simulink model "stoppuhr"  (R2021a)
settings: Solver=ode3  StartTime=0.0  StopTime=10.0  FixedStep=0.01  RelTol=1e-3
settings Model: Creator=Oceaner  LastModifiedBy=Oceaner

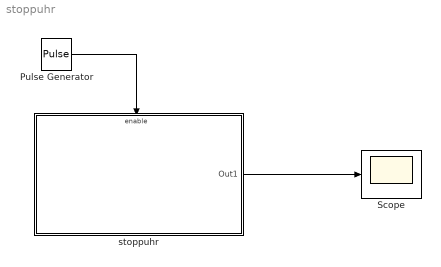
== system stoppuhr ==
  " stoppuhr" : Subsystem  TreatAsAtomicUnit=on
  Pulse Generator : DiscretePulseGenerator  PulseType=Time based  PulseWidth=50
  Scope : Scope
  wires:
  " stoppuhr"/1(Out1) -> Scope/1
  Pulse Generator/1 -> " stoppuhr"/Enable

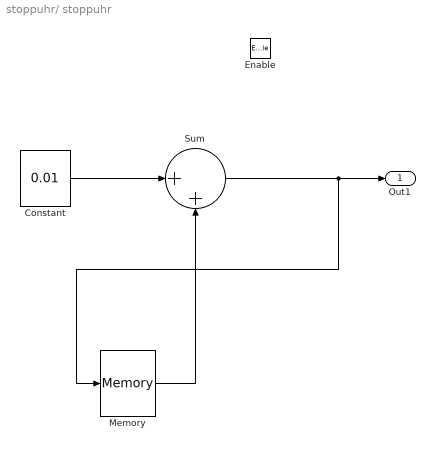
== system stoppuhr/ stoppuhr ==
  Enable : EnablePort
  Constant : Constant  Value=0.01
  Memory : Memory  InheritSampleTime=on
  Sum : Sum  Inputs=|++
  Out1 : Outport
  wires:
  Constant/1 -> Sum/1
  Memory/1 -> Sum/2
  Sum/1 -> Memory/1, Out1/1
